simulink library "controller_design_lib"  (Simulink 4.00)
settings Model: LastModifiedBy=bsaunder

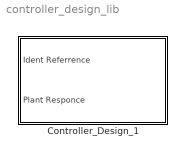
== system controller_design_lib ==
  Controller_Design_1 : Subsystem  mask(Controller Design Block){cntr_orders=[4 4 2 3], ctrObs_dyn=[3 0.9], refMdl_dyn=[3 0.9], Ts=0.05}
      mask prompts: cntr_orders "Controller Order [na nb nc nk]"; ctrObs_dyn "Controller observer dynamics [rise_Time_o damping_o]"; refMdl_dyn "Reference model dynamics  [rise_Time_m damping_m]"; Ts "Sample time"
      mask help: This block doesnt do much until the end of the simulation. During simulation termination this block calls a set of m-file functions that perform identification and controller synthesis. The results of which are saved on to the base workspace. If everything is successful then the results are also saved to a mat file with the name selected in this mask.
      settings: RTWFcnNameOpts=Auto  RTWFileNameOpts=Auto
      mask Display:
      | port_label('input', 1, 'P In');
      | port_label('input', 2, 'P Out');
      | 
      | plot([0.0 0.1 0.1 0.0; 0.1 0.1 0.0 0.0].*0.5+0.3, [0.0 0.0 0.1 0.1; 0.0 0.1 0.1 0.0]+0.15);
      | plot([0.0 0.1 0.1 0.0; 0.1 0.1 0.0 0.0].*0.5+0.3, [0.0 0.0 0.1 0.1; 0.0 0.1 0.1 0.0]+0.45);
      | plot([0.0 0.1 0.1 0.0; 0.1 0.1 0.0 0.0].*0.5+0.3, [0.0 0.0 0.1 0.1; 0.0 0.1 0.1 0.0]+0.75);
      | 
      | plot([0.00 0.16 0.20; 0.20 0.20 0.20].*0.5+0.4, [0.00 0.20 0.20; 0.20 0.20 0.15]+0.20);
      | plot([0.00 0.17 0.17; 0.20 0.20 0.20].*0.5+0.4, [0.10 0.13 0.07; 0.10 0.10 0.10]+0.40);
      | plot([0.00 0.16 0.20; 0.20 0.20 0.20].*0.5+0.4, [0.20 0.00 0.00; 0.00 0.00 0.05]+0.60);
      | 
      | plot([0.0 0.4 0.4 0.0; 0.4 0.4 0.0 0.0].*0.5+0.55, [0.0 0.0 0.4 0.4; 0.0 0.4 0.4 0.0]+0.3);
      | plot((sin([-pi:pi/90:0])).*0.1+0.7, (0.5+0.5.*cos([0:pi/90:pi])).*0.2+0.4);
      | 
      | plot([0.00 0.17 0.17; 0.20 0.20 0.20].*0.5+0.75, [0.10 0.13 0.07; 0.10 0.10 0.10]+0.40);
      | plot([0.0 0.1 0.1 0.0; 0.1 0.1 0.0 0.0]+0.85, [0.0 0.0 0.1 0.1; 0.0 0.1 0.1 0.0]+0.45);
      | plot([0.10 0.07 0.13; 0.10 0.10 0.10].*0.5+0.6, [0.00 0.07 0.07; 0.10 0.10 0.10]+0.2);
      | plot([0.00 0.25; 0.25 0.25]+0.65, [0.00 0.00; 0.00 0.25]+0.2);
      | 
      | text(0.7, 0.85, 'Controller Design', 'VerticalAlignment', 'middle', 'HorizontalAlignment', 'center');

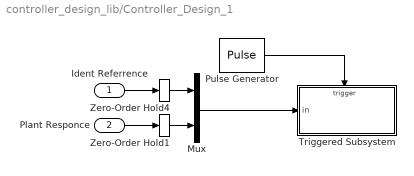
== system controller_design_lib/Controller_Design_1 ==
  Ident Referrence : Inport  Port=1  LatchInput=off
  Plant Responce : Inport  Port=2  LatchInput=off
  Mux : Mux  Inputs=2
  Pulse Generator : DiscretePulseGenerator  PulseType=Time-based  Amplitude=1  Period=2*Ts  PulseWidth=50  PhaseDelay=0  SampleTime=1
  Triggered Subsystem : Subsystem  TreatAsAtomicUnit=on
      settings: RTWFcnNameOpts=Auto  RTWFileNameOpts=Auto
  Zero-Order Hold1 : ZeroOrderHold  SampleTime=Ts
  Zero-Order Hold4 : ZeroOrderHold  SampleTime=Ts
  wires:
  Plant Responce/1 -> Zero-Order Hold1/1
  Ident Referrence/1 -> Zero-Order Hold4/1
  Mux/1 -> Triggered Subsystem/1(in)
  Pulse Generator/1 -> Triggered Subsystem/Trigger
  Zero-Order Hold4/1 -> Mux/1
  Zero-Order Hold1/1 -> Mux/2

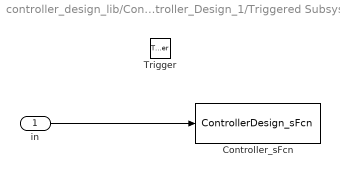
== system controller_design_lib/Controller_Design_1/Triggered Subsystem ==
  in : Inport  Port=1  LatchInput=off
  Trigger : TriggerPort  TriggerType=either  OutputDataType=auto
  Controller_sFcn : S-Function  FunctionName=ControllerDesign_sFcn  Parameters=cntr_orders, ctrObs_dyn, refMdl_dyn, Ts  PortCounts=[]  SFunctionModules=''
  wires:
  in/1 -> Controller_sFcn/1
